simulink model "auto_carelec"  (Simulink 6.0)
settings: Solver=ode23tb  StartTime=0.0  StopTime=3  MaxStep=0.001  RelTol=1e-3
InitFcn:
  | powericon('psbinitsys',bdroot);
libraries: powerlib2 x17, powerlib_extras x1
settings Model: Creator=The MathWorks Inc.  LastModifiedBy=batserve  ExtModeTrigMode=oneshot  ExtModeArmWhenConnect=off  ExtModeAutoUpdateStatusClock=off
settings DataIOCC: LimitDataPoints=off  SignalLoggingName=sigsOut
settings OptimizationCC: BooleanDataType=off
settings DebuggingCC: CheckExecutionContextPreStartOutputMsg=on  CheckExecutionContextRuntimeOutputMsg=on  SolverPrmCheckMsg=none
settings HardwareCC: TargetUnknown=on

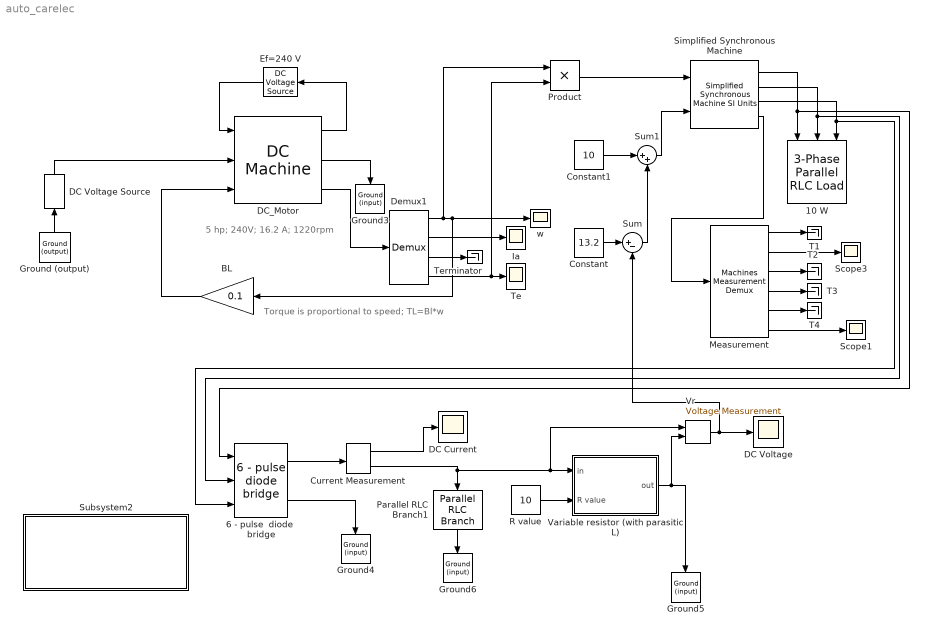
== system auto_carelec ==
  note: 5 hp; 240V; 16.2 A; 1220rpm
  note: Torque is proportional to speed; TL=Bl*w
  10 W : powerlib2/Elements/3-Phase Parallel RLC Load  Orientation=down  Vpp=20  fn=60  P3=1  QL3=0  QC3=0
  6 - pulse  diode  bridge : powerlib_extras/Three-Phase Library/6 - pulse  diode  bridge  Ron=0.01  Lon=10e-6  Vf=0.8  Rs=inf  Cs=100e-09
  BL : Gain  Orientation=left  Gain=0.1  SaturateOnIntegerOverflow=on
  Constant : Constant  Value=13.2
  Constant1 : Constant  Value=10
  Current Measurement : powerlib2/Measurements/Current Measurement  Tag=PoWeRsYsTeMmEaSuReMeNt  PhasorSimulation=off  OutputType=Magnitude  PSBOutputType=01  PSBequivalent=0
  DC Current : Scope
      settings: YMin=15  YMax=16.75
  DC Voltage : Scope
      settings: YMin=9.675  YMax=10.1
  DC Voltage Source : powerlib2/Electrical Sources/DC Voltage Source  Tag=PoWeRsYsTeMbLoCk  Orientation=up  V=160  mesure=None  PSBOutputType=1
  DC_Motor : powerlib2/Machines/DC Machine  RLa="[ 0.6  0.012]"  RLf="[ 240  120]"  Laf=1.8  J=1  Bm=0  Tf=0  w0=1  PSBOutputType=110
  Demux1 : Demux
  Ef=240 V : powerlib2/Electrical Sources/DC Voltage Source  Tag=PoWeRsYsTeMbLoCk  Orientation=left  V=240  mesure=None  PSBOutputType=1
  Ground (output) : powerlib2/Connectors/Ground (output)  Tag=PoWeRsYsTeMbLoCk  Orientation=up  PSBOutputType=1
  Ground{3..6} (4 alike) : powerlib2/Connectors/Ground (input)  Tag=PoWeRsYsTeMbLoCk  Orientation=down
  Ia : Scope
      settings: TickLabels=on  TimeRange=10  YMin=-50  YMax=400  SaveName=Ia  DataFormat=Array  MaxDataPoints=500000
  Measurement : powerlib2/Machines/Machines Measurement Demux  machType=Simplified synchronous  ssm1=on  ssm2=on  ssm3=on  ssm4=on  ssm5=on  ssm6=on  sm1=on  sm2=on  sm3=on  sm4=on  sm5=on  sm6=on  sm7=on  sm8=on  sm9=on  sm10=on  sm11=on  sm115=off  sm12=off  sm13=off  sm14=off  asm1=on  asm2=on  asm3=on  asm4=on  asm5=on  asm6=on  asm7=on  asm8=on  asm9=on  asm10=on  asm11=on  pmsm1=on  pmsm2=on  pmsm3=on  pmsm4=on  pmsm5=on  pmsm6=on  lastType=1
  Parallel RLC Branch1 : powerlib2/Elements/Parallel RLC Branch  Tag=PoWeRsYsTeMbLoCk  Orientation=down  a=100  b=inf  c=50e-06  mesure=None  PSBOutputType=1
  Product : Product  SaturateOnIntegerOverflow=on  InputSameDT=on
  R value : Constant  Value=10
  Scope1 : Scope
      settings: YMin=-17.5  YMax=17.5
  Scope3 : Scope
      settings: YMin=-17.5  YMax=17.5
  "Simplified Synchronous Machine " : powerlib2/Machines/Simplified Synchronous  Machine SI Units  Tag=PoWeRsYsTeMbLoCk  conType=3-wire Y  x1=[ 750, 20, 60 ]  x2=[ inf, 0, 3]  x3=[ 0.1, 2.15e-5 ]  x4="[ 0   0   0,0,0   0,0,0 ]"  PSBOutputType=1111  iounits=1  LoadFlowParameters=[1,0,0,0,0]
  Subsystem2 : Subsystem  Orientation=left  PropExecContextAcrossSSBoundary=on
      mask init:
      | % t1=matlabroot;
      | %cd(t1)
      | %test123=which('docE_file.html','-all');
      | %web(char(test123));
      settings: AttributesFormatString=\n
      settings: OpenFcn=|
      | docfile=which('auto_carelec.html','-all');
      | web(char(docfile));
      mask Display: disp('Double click\nhere for\n Model Information')
  Sum : Sum  Inputs=|+-  SaturateOnIntegerOverflow=on  InputSameDT=on
  Sum1 : Sum  Inputs=|++  SaturateOnIntegerOverflow=on  InputSameDT=on
  T{1..4} (4 alike) : Terminator
  Te : Scope
      settings: TickLabels=on  TimeRange=10  YMin=-100  YMax=800  SaveName=Tm  DataFormat=Array  MaxDataPoints=500000
  Terminator : Terminator
  "Variable resistor (with parasitic L) " : Subsystem  PropExecContextAcrossSSBoundary=on
      mask init:
      | [s1,s2,s3,s4,r1,r2,l1,l2,c1,c2,c3,c4,x1,x2,x3,x4] = powericon('Parallel RLC Branch',1,inf,0);
      mask Display: plot(s1-30,s2,s3+30,s4,r1,r2,l1,l2,c1,c2,c3,c4,x1,x2,x3,x4)
  Vr : powerlib2/Measurements/Voltage Measurement  Tag=PoWeRsYsTeMmEaSuReMeNt  PhasorSimulation=off  OutputType=Magnitude  PSBOutputType=0  PSBequivalent=0
  w : Scope
      settings: TickLabels=on  TimeRange=10  YMin=0  YMax=150  SaveName=w  DataFormat=Array  MaxDataPoints=500000
  wires:
  DC_Motor/3 -> Demux1/1
  DC_Motor/2 -> Ground3/1
  DC_Motor/1 -> Ef=240 V/1
  Demux1/3 -> Terminator/1
  Ef=240 V/1 -> DC_Motor/1
  Demux1/2 -> Ia/1
  Demux1/1 -> Product/1, BL/1, w/1
  DC Voltage Source/1 -> DC_Motor/2
  BL/1 -> DC_Motor/3
  Demux1/4 -> Te/1, Product/2
  Product/1 -> "Simplified Synchronous Machine "/1
  "Simplified Synchronous Machine "/4 -> Measurement/1
  "Simplified Synchronous Machine "/2 -> 10 W/2, 6 - pulse  diode  bridge/2
  "Simplified Synchronous Machine "/1 -> 10 W/1, 6 - pulse  diode  bridge/1
  Measurement/6 -> Scope1/1
  "Simplified Synchronous Machine "/3 -> 10 W/3, 6 - pulse  diode  bridge/3
  6 - pulse  diode  bridge/2 -> Ground4/1
  Parallel RLC Branch1/1 -> Ground6/1
  Measurement/2 -> Scope3/1
  Constant/1 -> Sum/1
  Constant1/1 -> Sum1/1
  Sum/1 -> Sum1/2
  Sum1/1 -> "Simplified Synchronous Machine "/2
  Vr/1 -> DC Voltage/1, Sum/2
  6 - pulse  diode  bridge/1 -> Current Measurement/1
  Current Measurement/2 -> Parallel RLC Branch1/1, "Variable resistor (with parasitic L) "/1(in), Vr/1
  Current Measurement/1 -> DC Current/1
  Ground (output)/1 -> DC Voltage Source/1
  R value/1 -> "Variable resistor (with parasitic L) "/2(R value)
  "Variable resistor (with parasitic L) "/1(out) -> Ground5/1, Vr/2
  Measurement/1 -> T1/1
  Measurement/3 -> T2/1
  Measurement/4 -> T3/1
  Measurement/5 -> T4/1

== system auto_carelec/Subsystem2 ==

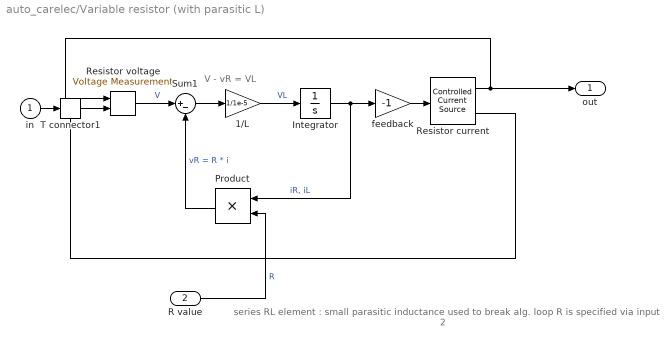
== system auto_carelec/Variable resistor (with parasitic L)  ==
  note: V - vR = VL
  note: series RL element : small parasitic inductance used to break alg. loop
      | R is specified via input 2
  in : Inport  Port=1  LatchInput=off
  R value : Inport  Port=2  LatchInput=off
  1/L : Gain  Gain=1/1e-5  SaturateOnIntegerOverflow=on
  Integrator : Integrator  ZeroCross=off
  Product : Product  Orientation=left  SaturateOnIntegerOverflow=on  InputSameDT=on
  Resistor current : powerlib2/Electrical Sources/Controlled Current Source  Tag=PoWeRsYsTeMbLoCk  Description=source block  initsrc=on  srctyp=DC  ia=0  iph=0  freq=0  mesure=None  PSBOutputType=11
  Resistor voltage : powerlib2/Measurements/Voltage Measurement  Tag=PoWeRsYsTeMmEaSuReMeNt  PSBOutputType=0  PSBequivalent=0
  Sum1 : Sum  Inputs=|+-  SaturateOnIntegerOverflow=on  InputSameDT=on
  T connector1 : powerlib2/Connectors/T connector  Tag=PoWeRsYsTeMbLoCk  PSBOutputType=1
  feedback : Gain  Gain=-1  SaturateOnIntegerOverflow=on
  out : Outport
  wires:
  Resistor current/1 -> out/1, Resistor voltage/1
  in/1 -> T connector1/1
  Sum1/1 -> 1/L/1
  Resistor current/2 -> T connector1/Enable
  T connector1/1 -> Resistor voltage/2
  Integrator/1 -> Product/1, feedback/1  "iR, iL"
  1/L/1 -> Integrator/1  "VL"
  Resistor voltage/1 -> Sum1/1  "V"
  R value/1 -> Product/2  "R"
  Product/1 -> Sum1/2  "vR = R * i"
  feedback/1 -> Resistor current/1
